simulink model "plant_test"  (R2023b)
settings: Solver=VariableStepAuto  StartTime=0.0  StopTime=t_end  RelTol=1e-3
undefined symbols (not defined in the file): dt, sysc, ue, w, x0, xe
libraries: fl_lib x10, nesl_utility x4
(part 3 of 3)

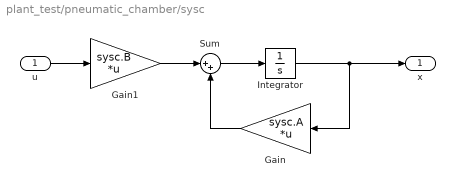
== system plant_test/pneumatic_chamber/sysc ==
  u : Inport
  Gain : Gain  Gain=sysc.A  Multiplication=Matrix(K*u)
  Gain1 : Gain  Gain=sysc.B  Multiplication=Matrix(K*u)
  Integrator : Integrator  InitialCondition=x0
  Sum : Sum  Inputs=|++
  x : Outport
  wires:
  Sum/1 -> Integrator/1
  u/1 -> Gain1/1
  Gain1/1 -> Sum/1
  Gain/1 -> Sum/2
  Integrator/1 -> x/1, Gain/1

== system plant_test/signal_generator/impulse ==
  Step1 : Step  Time=1e-3  Before=1e-3  After=0  SampleTime=0
  target : Outport
  wires:
  Step1/1 -> target/1

== system plant_test/signal_generator/sine ==
  Sine Wave1 : Sin  Amplitude=1e-6  Frequency=w  SampleTime=0
  target : Outport
  wires:
  Sine Wave1/1 -> target/1

== system plant_test/signal_generator/zero ==
  Constant : Constant  Value=0
  target : Outport
  wires:
  Constant/1 -> target/1

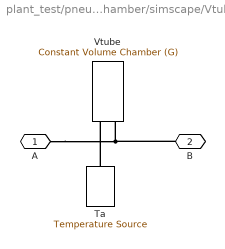
== system plant_test/pneumatic_chamber/simscape/Vtube ==
  Ta : fl_lib/Thermal/Thermal Sources/Temperature Source  temperature=param.Ta K
  Vtube : fl_lib/Gas/Elements/Constant Volume Chamber (G)  volume=param.Vtube m^3  num_ports=foundation.enum.num_ports.one  area_A=0.01 m^2  area_B=0.01 m^2  area_C=0.01 m^2  area_D=0.01 m^2  p_I_specify=on  p_I_priority=High  p_I=x0(1) Pa  p_I_nominal_specify=off  p_I_nominal_unit=MPa  p_I_nominal_value=1  T_I_specify=off  T_I_priority=High  T_I=293.15 K  T_I_nominal_specify=off  T_I_nominal_unit=K  T_I_nominal_value=1  rho_I_specify=off  rho_I_priority=None  rho_I=1.2 kg/m^3  rho_I_nominal_specify=off  rho_I_nominal_unit=kg/m^3  rho_I_nominal_value=1
      settings: InternalSimscapePortConfiguration="{\"Bottom\":[],\"Left\":[{\"id\":\"A\",\"label\":\"A\",\"type\":\"foundation.gas.gas\"},{\"id\":\"H\",\"label\":\"H\",\"type\":\"foundation.thermal.thermal\"}],\"Right\":[],\"Top\":[]}"
  A : PMIOPort  Side=Left
  B : PMIOPort  Port=2  Side=Right
  connections:
  A/RConn1 -- B/RConn1 -- Vtube/LConn1
  Ta/LConn1 -- Vtube/LConn2

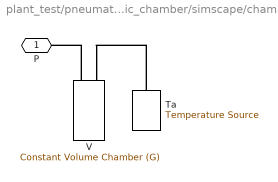
== system plant_test/pneumatic_chamber/simscape/chamber ==
  Ta : fl_lib/Thermal/Thermal Sources/Temperature Source  temperature=param.Ta K
  V : fl_lib/Gas/Elements/Constant Volume Chamber (G)  volume=param.V m^3  num_ports=foundation.enum.num_ports.one  area_A=0.01 m^2  area_B=0.01 m^2  area_C=0.01 m^2  area_D=0.01 m^2  p_I_specify=on  p_I_priority=High  p_I=x0(1) Pa  p_I_nominal_specify=off  p_I_nominal_unit=MPa  p_I_nominal_value=1  T_I_specify=off  T_I_priority=High  T_I=293.15 K  T_I_nominal_specify=off  T_I_nominal_unit=K  T_I_nominal_value=1  rho_I_specify=off  rho_I_priority=None  rho_I=1.2 kg/m^3  rho_I_nominal_specify=off  rho_I_nominal_unit=kg/m^3  rho_I_nominal_value=1
      settings: InternalSimscapePortConfiguration="{\"Bottom\":[],\"Left\":[{\"id\":\"A\",\"label\":\"A\",\"type\":\"foundation.gas.gas\"},{\"id\":\"H\",\"label\":\"H\",\"type\":\"foundation.thermal.thermal\"}],\"Right\":[],\"Top\":[]}"
  P : PMIOPort  Side=Left
  connections:
  Ta/LConn1 -- V/LConn2
  V/LConn1 -- P/RConn1

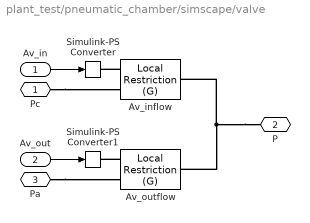
== system plant_test/pneumatic_chamber/simscape/valve ==
  Av_in : Inport
  Av_out : Inport  Port=2
  Av_inflow : fl_lib/Gas/Elements/Local Restriction (G)  restriction_type=foundation.enum.restriction_type.variable  restriction_area=1e-3 m^2  min_area=eps m^2  max_area=param.Av m^2  area=0.01 m^2  Cd=0.8975  B_lam=0.999
      settings: InternalSimscapePortConfiguration="{\"Bottom\":[],\"Left\":[{\"id\":\"A\",\"label\":\"A\",\"type\":\"foundation.gas.gas\"},{\"id\":\"area_in\",\"label\":\"AR\",\"type\":\"input\"}],\"Right\":[{\"id\":\"B\",\"label\":\"B\",\"type\":\"foundation.gas.gas\"}],\"Top\":[]}"
  Av_outflow : fl_lib/Gas/Elements/Local Restriction (G)  restriction_type=foundation.enum.restriction_type.variable  restriction_area=1e-3 m^2  min_area=eps m^2  max_area=param.Av m^2  area=0.01 m^2  Cd=0.8975  B_lam=0.999
      settings: InternalSimscapePortConfiguration="{\"Bottom\":[],\"Left\":[{\"id\":\"A\",\"label\":\"A\",\"type\":\"foundation.gas.gas\"},{\"id\":\"area_in\",\"label\":\"AR\",\"type\":\"input\"}],\"Right\":[{\"id\":\"B\",\"label\":\"B\",\"type\":\"foundation.gas.gas\"}],\"Top\":[]}"
  Simulink-PS Converter : nesl_utility/Simulink-PS Converter  PhysicalDomain=network_engine_domain  SubClassName=ps_input  LeftPortType=input  RightPortType=output  PseudoPeriodic=off  Frequencies=[]  NoiseDistribution=none  NoiseParameters=[]  Unit=1  AffineConversion=off  FilteringAndDerivatives=provide  SimscapeFilterOrder=1  InputFilterTimeConstant=0.001  UdotUserProvided=0
  Simulink-PS Converter1 : nesl_utility/Simulink-PS Converter  PhysicalDomain=network_engine_domain  SubClassName=ps_input  LeftPortType=input  RightPortType=output  PseudoPeriodic=off  Frequencies=[]  NoiseDistribution=none  NoiseParameters=[]  Unit=1  AffineConversion=off  FilteringAndDerivatives=provide  SimscapeFilterOrder=1  InputFilterTimeConstant=0.001  UdotUserProvided=0
  Pc : PMIOPort  Side=Left
  P : PMIOPort  Port=2  Side=Right
  Pa : PMIOPort  Port=3  Side=Right
  wires:
  Av_in/1 -> Simulink-PS Converter/1
  Av_out/1 -> Simulink-PS Converter1/1
  connections:
  Pc/RConn1 -- Av_inflow/LConn1
  Av_inflow/LConn2 -- Simulink-PS Converter/RConn1
  Pa/RConn1 -- Av_outflow/LConn1
  Av_outflow/LConn2 -- Simulink-PS Converter1/RConn1
  P/RConn1 -- Av_outflow/RConn1 -- Av_inflow/RConn1

== matlab function plant_test/pneumatic_chamber/ode/MATLAB Function ==
  data: x input size=param.xdim; u input size=param.udim; dxdt output size=param.xdim; param parameter
function dxdt = ode(x,u,param)
    dxdt = plant_ode(0,x,u,param);
end

== matlab function plant_test/input_transform/udim==2/valve ==
  data: mu input size=1; x input size=1; Av output size=2; param parameter
function Av = valve(mu,x,param)
    Pa = param.Pa;
    Ps = param.Ps;
    alpha_in = param.alpha_in;
    alpha_out = param.alpha_out;

    P = x(1);

    if mu > 0
        Av = [mu/(alpha_in*phi(Ps,P,param));0];
    elseif mu < 0
        Av = [0;-mu/(alpha_out*phi(P,Pa,param))];
    else
        Av = [0;0];
    end
end

function ret = phi(P1,P2,param)
    R = param.R;
    Ta = param.Ta;
    k = param.k;
    Pcr = (2/(k + 1))^(k/(k - 1)); % critical pressure ratio (-)
    C1 = sqrt(k*(2/(k + 1))^((k + 1)/(k - 1)));
    C2 = sqrt(2*k/(k - 1));

    if (P2/P1) < Pcr
        ret = C1*(P1/sqrt(R*Ta));
    elseif (P2/P1) < 1
        ret = C2*(P1/sqrt(R*Ta))*(P2/P1)^(1/k)*sqrt(1 - (P2/P1)^((k - 1)/k));
    elseif (P2/P1) < (1/Pcr)
        ret = -C2*(P2/sqrt(R*Ta))*(P1/P2)^(1/k)*sqrt(1 - (P1/P2)^((k - 1)/k));
    else
        ret = -C1*(P2/sqrt(R*Ta));
    end
end
